simulink model "TorqueVectoring"  (R2024b)
settings: configuration reference "STM32H7_Config" (kept outside this file)
undefined symbols (not defined in the file): FStaticWeightFront, FStaticWeightRear, IYawInertia, lTrackWidth, lWheelbase, mCarMass, MMotorMaxAllowed, MMotorMinAllowed, MNominal, rGearboxRatio, rTyreRadius, tTorqueVectoringErrorCorrection, zCogHeight
libraries: simulink x10
settings Model: DataDictionary=Master_Dictionary.sldd  EnableAccessToBaseWorkspace=off  Creator=torni  LastModifiedBy=William
settings ConfigSetRef: SourceName=STM32H7_Config

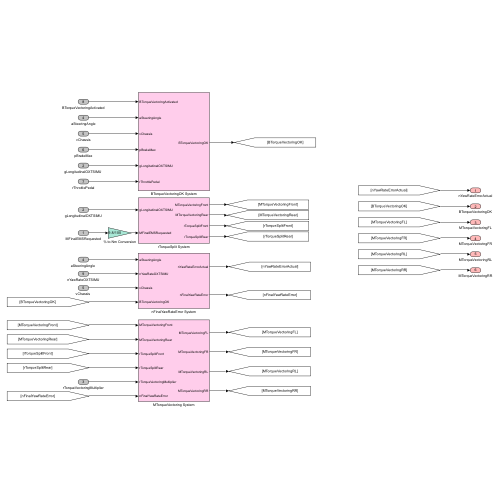
[thumbnail: Simulink's stored preview of the top-level diagram]
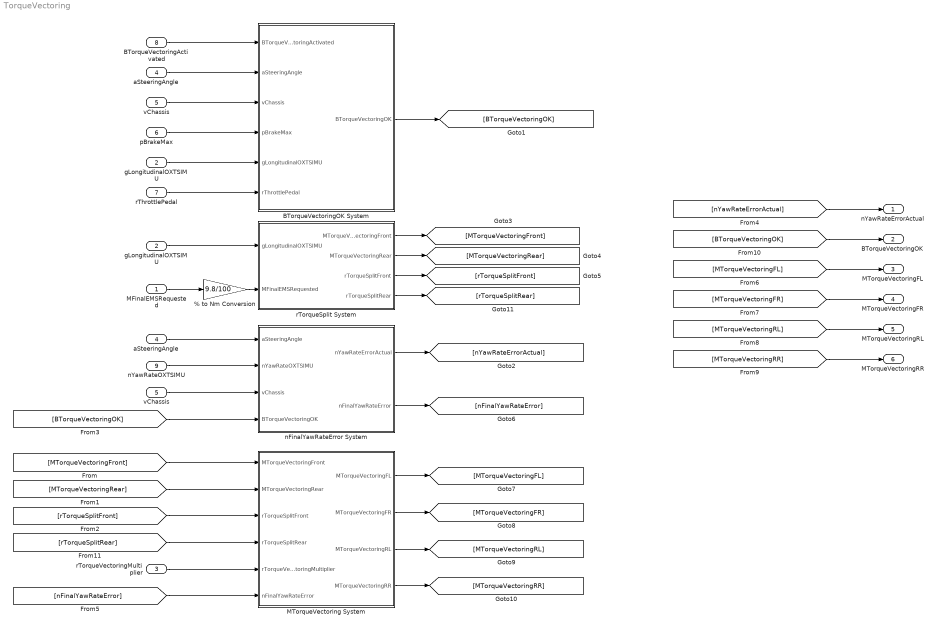
== system TorqueVectoring ==
  MFinalEMSRequested : Inport  OutDataTypeStr=double
  gLongitudinalOXTSIMU : Inport  Port=2  OutDataTypeStr=double
  rTorqueVectoringMultiplier : Inport  Port=3  OutDataTypeStr=double
  aSteeringAngle : Inport  Port=4  OutDataTypeStr=double
  vChassis : Inport  Port=5  OutDataTypeStr=double
  pBrakeMax : Inport  Port=6  OutDataTypeStr=double
  rThrottlePedal : Inport  Port=7  OutDataTypeStr=double
  BTorqueVectoringActivated : Inport  Port=8  OutDataTypeStr=boolean
  nYawRateOXTSIMU : Inport  Port=9  OutDataTypeStr=double
  % to Nm Conversion : Gain  Gain=9.8/100
  BTorqueVectoringOK System : Subsystem
  MTorqueVectoring System : Subsystem
  "aSteeringAngle " : InportShadow  Port=4  OutDataTypeStr=double
  "gLongitudinalOXTSIMU " : InportShadow  Port=2  OutDataTypeStr=double
  nFinalYawRateError System : Subsystem
  rTorqueSplit System : Subsystem
  "vChassis " : InportShadow  Port=5  OutDataTypeStr=double
  nYawRateErrorActual : Outport  OutDataTypeStr=double  VectorParamsAs1DForOutWhenUnconnected=off
  BTorqueVectoringOK : Outport  Port=2  OutDataTypeStr=boolean  VectorParamsAs1DForOutWhenUnconnected=off
  MTorqueVectoringFL : Outport  Port=3  OutDataTypeStr=double  VectorParamsAs1DForOutWhenUnconnected=off
  MTorqueVectoringFR : Outport  Port=4  OutDataTypeStr=double  VectorParamsAs1DForOutWhenUnconnected=off
  MTorqueVectoringRL : Outport  Port=5  OutDataTypeStr=double  VectorParamsAs1DForOutWhenUnconnected=off
  MTorqueVectoringRR : Outport  Port=6  OutDataTypeStr=double  VectorParamsAs1DForOutWhenUnconnected=off
  wires:
  rTorqueSplit System/2(MTorqueVectoringRear) -> [MTorqueVectoringRear]
  gLongitudinalOXTSIMU/1 -> rTorqueSplit System/1(gLongitudinalOXTSIMU)
  % to Nm Conversion/1 -> rTorqueSplit System/2(MFinalEMSRequested)
  MFinalEMSRequested/1 -> % to Nm Conversion/1
  rTorqueSplit System/1(MTorqueVectoringFront) -> [MTorqueVectoringFront]
  rTorqueSplit System/3(rTorqueSplitFront) -> [rTorqueSplitFront]
  [MTorqueVectoringFront] -> MTorqueVectoring System/1(MTorqueVectoringFront)
  [rTorqueSplitFront] -> MTorqueVectoring System/3(rTorqueSplitFront)
  BTorqueVectoringActivated/1 -> BTorqueVectoringOK System/1(BTorqueVectoringActivated)
  aSteeringAngle/1 -> BTorqueVectoringOK System/2(aSteeringAngle)
  vChassis/1 -> BTorqueVectoringOK System/3(vChassis)
  pBrakeMax/1 -> BTorqueVectoringOK System/4(pBrakeMax)
  "gLongitudinalOXTSIMU "/1 -> BTorqueVectoringOK System/5(gLongitudinalOXTSIMU)
  rThrottlePedal/1 -> BTorqueVectoringOK System/6(rThrottlePedal)
  BTorqueVectoringOK System/1(BTorqueVectoringOK) -> [BTorqueVectoringOK]
  rTorqueVectoringMultiplier/1 -> MTorqueVectoring System/5(rTorqueVectoringMultiplier)
  "aSteeringAngle "/1 -> nFinalYawRateError System/1(aSteeringAngle)
  nYawRateOXTSIMU/1 -> nFinalYawRateError System/2(nYawRateOXTSIMU)
  "vChassis "/1 -> nFinalYawRateError System/3(vChassis)
  [BTorqueVectoringOK] -> nFinalYawRateError System/4(BTorqueVectoringOK)
  nFinalYawRateError System/1(nYawRateErrorActual) -> [nYawRateErrorActual]
  nFinalYawRateError System/2(nFinalYawRateError) -> [nFinalYawRateError]
  [MTorqueVectoringRear] -> MTorqueVectoring System/2(MTorqueVectoringRear)
  [nFinalYawRateError] -> MTorqueVectoring System/6(nFinalYawRateError)
  MTorqueVectoring System/1(MTorqueVectoringFL) -> [MTorqueVectoringFL]
  MTorqueVectoring System/2(MTorqueVectoringFR) -> [MTorqueVectoringFR]
  MTorqueVectoring System/3(MTorqueVectoringRL) -> [MTorqueVectoringRL]
  MTorqueVectoring System/4(MTorqueVectoringRR) -> [MTorqueVectoringRR]
  [nYawRateErrorActual] -> nYawRateErrorActual/1
  [BTorqueVectoringOK] -> BTorqueVectoringOK/1
  [MTorqueVectoringFL] -> MTorqueVectoringFL/1
  [MTorqueVectoringFR] -> MTorqueVectoringFR/1
  [MTorqueVectoringRL] -> MTorqueVectoringRL/1
  [MTorqueVectoringRR] -> MTorqueVectoringRR/1
  rTorqueSplit System/4(rTorqueSplitRear) -> [rTorqueSplitRear]
  [rTorqueSplitRear] -> MTorqueVectoring System/4(rTorqueSplitRear)

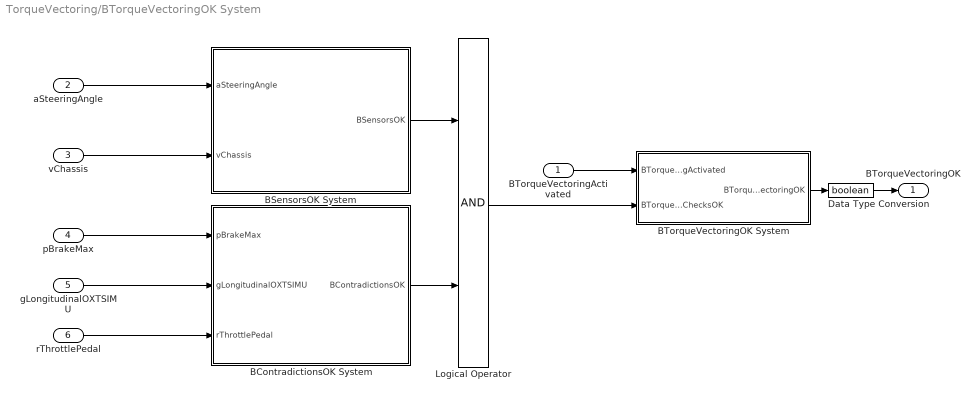
== system TorqueVectoring/BTorqueVectoringOK System ==
  BTorqueVectoringActivated : Inport  OutDataTypeStr=boolean
  aSteeringAngle : Inport  Port=2  OutDataTypeStr=double
  vChassis : Inport  Port=3  OutDataTypeStr=double
  pBrakeMax : Inport  Port=4  OutDataTypeStr=double
  gLongitudinalOXTSIMU : Inport  Port=5  OutDataTypeStr=double
  rThrottlePedal : Inport  Port=6  OutDataTypeStr=double
  BContradictionsOK System : Subsystem
  BSensorsOK System : Subsystem
  BTorqueVectoringOK System : Stateflow chart  TreatAsAtomicUnit=on
  Data Type Conversion : DataTypeConversion  OutDataTypeStr=boolean  SaturateOnIntegerOverflow=off  RndMeth=Floor
  Logical Operator : Logic  AllPortsSameDT=off  OutDataTypeStr=boolean
  BTorqueVectoringOK : Outport  OutDataTypeStr=boolean  VectorParamsAs1DForOutWhenUnconnected=off
  wires:
  pBrakeMax/1 -> BContradictionsOK System/1(pBrakeMax)
  rThrottlePedal/1 -> BContradictionsOK System/3(rThrottlePedal)
  Logical Operator/1 -> BTorqueVectoringOK System/2(BTorqueVectoringChecksOK)
  BTorqueVectoringOK System/1(BTorqueVectoringOK) -> Data Type Conversion/1
  BContradictionsOK System/1(BContradictionsOK) -> Logical Operator/2
  gLongitudinalOXTSIMU/1 -> BContradictionsOK System/2(gLongitudinalOXTSIMU)
  vChassis/1 -> BSensorsOK System/2(vChassis)
  BSensorsOK System/1(BSensorsOK) -> Logical Operator/1
  aSteeringAngle/1 -> BSensorsOK System/1(aSteeringAngle)
  BTorqueVectoringActivated/1 -> BTorqueVectoringOK System/1(BTorqueVectoringActivated)
  Data Type Conversion/1 -> BTorqueVectoringOK/1

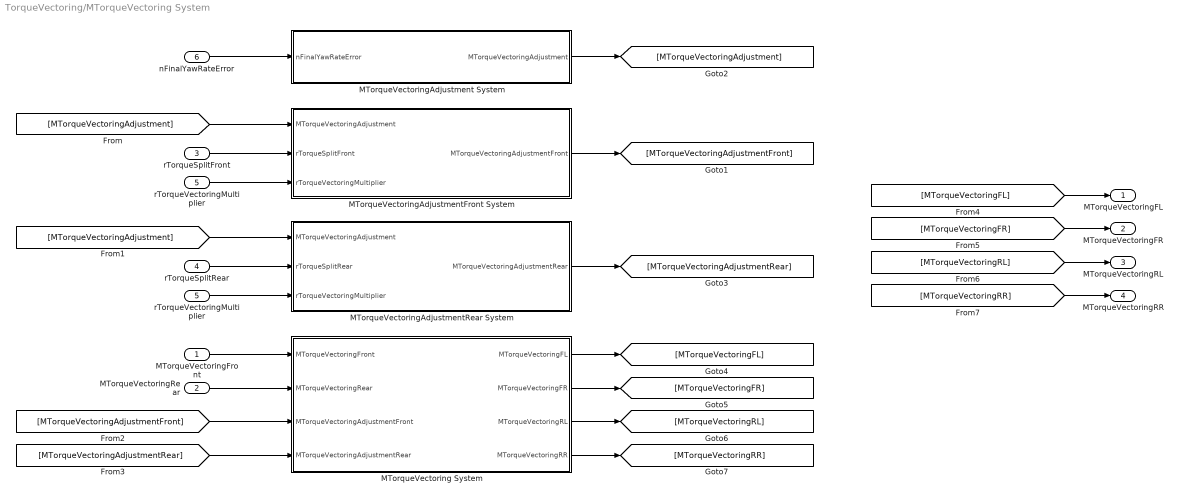
== system TorqueVectoring/MTorqueVectoring System ==
  MTorqueVectoringFront : Inport
  MTorqueVectoringRear : Inport  Port=2
  rTorqueSplitFront : Inport  Port=3  OutDataTypeStr=double
  rTorqueSplitRear : Inport  Port=4  OutDataTypeStr=double
  rTorqueVectoringMultiplier : Inport  Port=5  OutDataTypeStr=double
  nFinalYawRateError : Inport  Port=6  OutDataTypeStr=double
  MTorqueVectoring System : Subsystem
  MTorqueVectoringAdjustment System : Subsystem
  MTorqueVectoringAdjustmentFront System : Subsystem
  MTorqueVectoringAdjustmentRear System : Subsystem
  "rTorqueVectoringMultiplier " : InportShadow  Port=5  OutDataTypeStr=double
  MTorqueVectoringFL : Outport  OutDataTypeStr=double  VectorParamsAs1DForOutWhenUnconnected=off
  MTorqueVectoringFR : Outport  Port=2  OutDataTypeStr=double  VectorParamsAs1DForOutWhenUnconnected=off
  MTorqueVectoringRL : Outport  Port=3  OutDataTypeStr=double  VectorParamsAs1DForOutWhenUnconnected=off
  MTorqueVectoringRR : Outport  Port=4  OutDataTypeStr=double  VectorParamsAs1DForOutWhenUnconnected=off
  wires:
  nFinalYawRateError/1 -> MTorqueVectoringAdjustment System/1(nFinalYawRateError)
  MTorqueVectoringAdjustment System/1(MTorqueVectoringAdjustment) -> [MTorqueVectoringAdjustment]
  rTorqueSplitFront/1 -> MTorqueVectoringAdjustmentFront System/2(rTorqueSplitFront)
  [MTorqueVectoringAdjustment] -> MTorqueVectoringAdjustmentFront System/1(MTorqueVectoringAdjustment)
  rTorqueVectoringMultiplier/1 -> MTorqueVectoringAdjustmentFront System/3(rTorqueVectoringMultiplier)
  MTorqueVectoringAdjustmentFront System/1(MTorqueVectoringAdjustmentFront) -> [MTorqueVectoringAdjustmentFront]
  [MTorqueVectoringAdjustment] -> MTorqueVectoringAdjustmentRear System/1(MTorqueVectoringAdjustment)
  rTorqueSplitRear/1 -> MTorqueVectoringAdjustmentRear System/2(rTorqueSplitRear)
  "rTorqueVectoringMultiplier "/1 -> MTorqueVectoringAdjustmentRear System/3(rTorqueVectoringMultiplier)
  MTorqueVectoringAdjustmentRear System/1(MTorqueVectoringAdjustmentRear) -> [MTorqueVectoringAdjustmentRear]
  MTorqueVectoringFront/1 -> MTorqueVectoring System/1(MTorqueVectoringFront)
  MTorqueVectoringRear/1 -> MTorqueVectoring System/2(MTorqueVectoringRear)
  [MTorqueVectoringAdjustmentFront] -> MTorqueVectoring System/3(MTorqueVectoringAdjustmentFront)
  [MTorqueVectoringAdjustmentRear] -> MTorqueVectoring System/4(MTorqueVectoringAdjustmentRear)
  MTorqueVectoring System/1(MTorqueVectoringFL) -> [MTorqueVectoringFL]
  MTorqueVectoring System/2(MTorqueVectoringFR) -> [MTorqueVectoringFR]
  MTorqueVectoring System/3(MTorqueVectoringRL) -> [MTorqueVectoringRL]
  MTorqueVectoring System/4(MTorqueVectoringRR) -> [MTorqueVectoringRR]
  [MTorqueVectoringFL] -> MTorqueVectoringFL/1
  [MTorqueVectoringFR] -> MTorqueVectoringFR/1
  [MTorqueVectoringRL] -> MTorqueVectoringRL/1
  [MTorqueVectoringRR] -> MTorqueVectoringRR/1

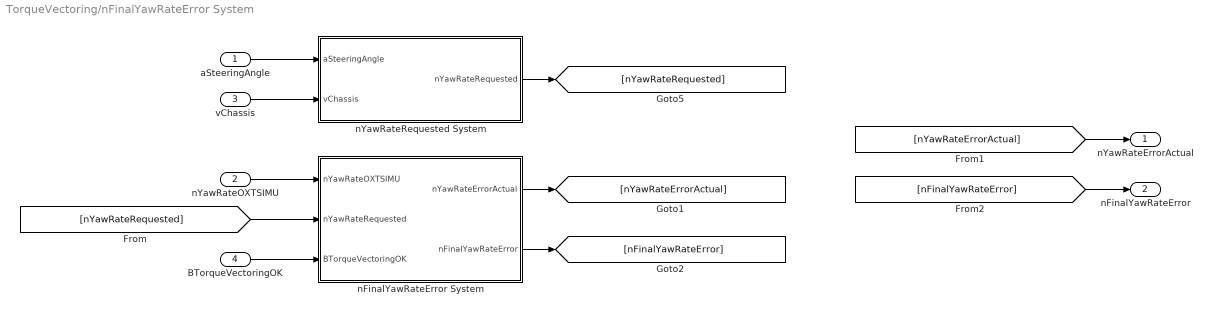
== system TorqueVectoring/nFinalYawRateError System ==
  aSteeringAngle : Inport  OutDataTypeStr=double
  nYawRateOXTSIMU : Inport  Port=2  OutDataTypeStr=double
  vChassis : Inport  Port=3  OutDataTypeStr=double
  BTorqueVectoringOK : Inport  Port=4  OutDataTypeStr=boolean
  nFinalYawRateError System : Subsystem
  nYawRateRequested System : Subsystem
  nYawRateErrorActual : Outport  OutDataTypeStr=double  VectorParamsAs1DForOutWhenUnconnected=off
  nFinalYawRateError : Outport  Port=2  OutDataTypeStr=double  VectorParamsAs1DForOutWhenUnconnected=off
  wires:
  aSteeringAngle/1 -> nYawRateRequested System/1(aSteeringAngle)
  vChassis/1 -> nYawRateRequested System/2(vChassis)
  nYawRateRequested System/1(nYawRateRequested) -> [nYawRateRequested]
  nYawRateOXTSIMU/1 -> nFinalYawRateError System/1(nYawRateOXTSIMU)
  [nYawRateRequested] -> nFinalYawRateError System/2(nYawRateRequested)
  BTorqueVectoringOK/1 -> nFinalYawRateError System/3(BTorqueVectoringOK)
  nFinalYawRateError System/1(nYawRateErrorActual) -> [nYawRateErrorActual]
  nFinalYawRateError System/2(nFinalYawRateError) -> [nFinalYawRateError]
  [nYawRateErrorActual] -> nYawRateErrorActual/1
  [nFinalYawRateError] -> nFinalYawRateError/1

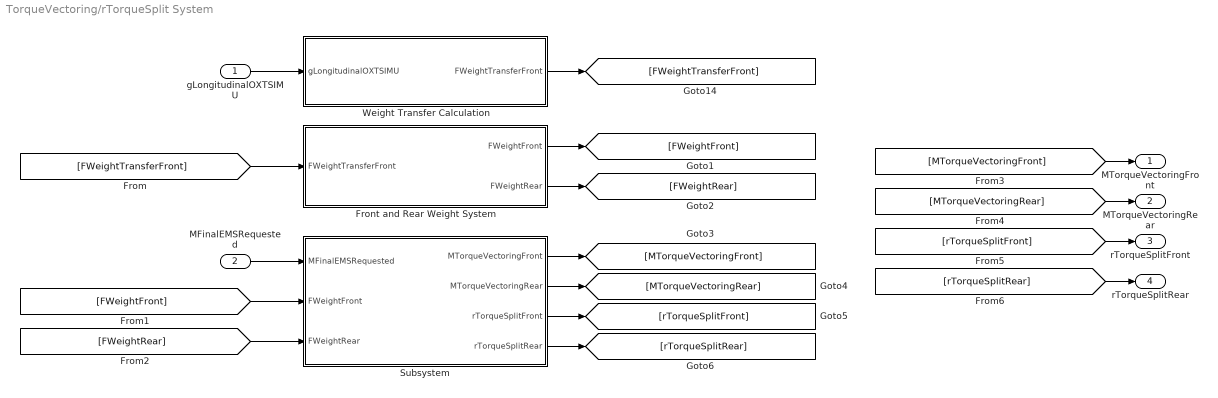
== system TorqueVectoring/rTorqueSplit System ==
  gLongitudinalOXTSIMU : Inport  OutDataTypeStr=double
  MFinalEMSRequested : Inport  Port=2  OutDataTypeStr=double
  Front and Rear Weight System : Subsystem
  Subsystem : Subsystem
  Weight Transfer Calculation : Subsystem
  MTorqueVectoringFront : Outport  OutDataTypeStr=double  VectorParamsAs1DForOutWhenUnconnected=off
  MTorqueVectoringRear : Outport  Port=2  OutDataTypeStr=double  VectorParamsAs1DForOutWhenUnconnected=off
  rTorqueSplitFront : Outport  Port=3  OutDataTypeStr=double  VectorParamsAs1DForOutWhenUnconnected=off
  rTorqueSplitRear : Outport  Port=4  OutDataTypeStr=double  VectorParamsAs1DForOutWhenUnconnected=off
  wires:
  Weight Transfer Calculation/1(FWeightTransferFront) -> [FWeightTransferFront]
  gLongitudinalOXTSIMU/1 -> Weight Transfer Calculation/1(gLongitudinalOXTSIMU)
  [FWeightTransferFront] -> Front and Rear Weight System/1(FWeightTransferFront)
  Front and Rear Weight System/1(FWeightFront) -> [FWeightFront]
  Front and Rear Weight System/2(FWeightRear) -> [FWeightRear]
  MFinalEMSRequested/1 -> Subsystem/1(MFinalEMSRequested)
  [FWeightFront] -> Subsystem/2(FWeightFront)
  [FWeightRear] -> Subsystem/3(FWeightRear)
  Subsystem/1(MTorqueVectoringFront) -> [MTorqueVectoringFront]
  Subsystem/2(MTorqueVectoringRear) -> [MTorqueVectoringRear]
  Subsystem/3(rTorqueSplitFront) -> [rTorqueSplitFront]
  [MTorqueVectoringFront] -> MTorqueVectoringFront/1
  [MTorqueVectoringRear] -> MTorqueVectoringRear/1
  [rTorqueSplitFront] -> rTorqueSplitFront/1
  Subsystem/4(rTorqueSplitRear) -> [rTorqueSplitRear]
  [rTorqueSplitRear] -> rTorqueSplitRear/1

== system TorqueVectoring/BTorqueVectoringOK System/BContradictionsOK System ==
  pBrakeMax : Inport  OutDataTypeStr=double
  gLongitudinalOXTSIMU : Inport  Port=2  OutDataTypeStr=double
  rThrottlePedal : Inport  Port=3  OutDataTypeStr=double
  Brake Contradiction : Subsystem
  Data Type Conversion : DataTypeConversion  OutDataTypeStr=boolean  SaturateOnIntegerOverflow=off  RndMeth=Floor
  Logical Operator : Logic  AllPortsSameDT=off  OutDataTypeStr=boolean
  Throttle Contradiction : Subsystem
  BContradictionsOK : Outport  OutDataTypeStr=boolean  VectorParamsAs1DForOutWhenUnconnected=off
  wires:
  Throttle Contradiction/1(BThrottleContradictionOK) -> Logical Operator/2
  Brake Contradiction/1(BBrakeContradictionOK) -> Logical Operator/1
  Logical Operator/1 -> Data Type Conversion/1
  pBrakeMax/1 -> Brake Contradiction/1(pBrakeMax)
  gLongitudinalOXTSIMU/1 -> Brake Contradiction/2(gLongitudinalOXTSIMU), Throttle Contradiction/1(gLongitudinalBoschIMU)
  rThrottlePedal/1 -> Throttle Contradiction/2(rThrottlePedal)
  Data Type Conversion/1 -> BContradictionsOK/1

== system TorqueVectoring/BTorqueVectoringOK System/BSensorsOK System ==
  aSteeringAngle : Inport  OutDataTypeStr=double
  vChassis : Inport  Port=2  OutDataTypeStr=double
  BSteeringAngleOK System : Subsystem
  BVelocityOK System : Subsystem
  Logical Operator : Logic  AllPortsSameDT=off  OutDataTypeStr=boolean
  BSensorsOK : Outport  OutDataTypeStr=boolean  VectorParamsAs1DForOutWhenUnconnected=off
  wires:
  BVelocityOK System/1(BVelocityOK) -> Logical Operator/1
  BSteeringAngleOK System/1(BSteeringAngleOK) -> Logical Operator/2
  Logical Operator/1 -> BSensorsOK/1
  vChassis/1 -> BVelocityOK System/1(vChassis)
  aSteeringAngle/1 -> BSteeringAngleOK System/1(aSteeringAngle)

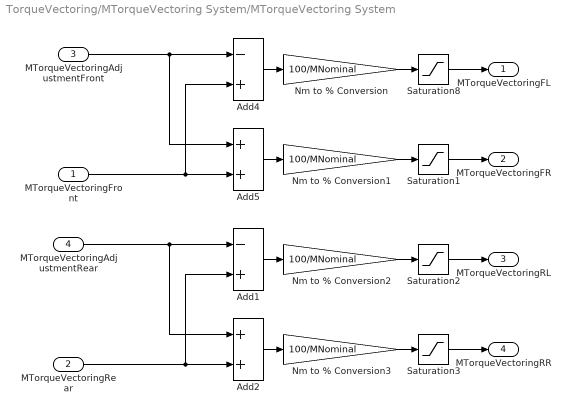
== system TorqueVectoring/MTorqueVectoring System/MTorqueVectoring System ==
  MTorqueVectoringFront : Inport  OutDataTypeStr=double
  MTorqueVectoringRear : Inport  Port=2  OutDataTypeStr=double
  MTorqueVectoringAdjustmentFront : Inport  Port=3  OutDataTypeStr=double
  MTorqueVectoringAdjustmentRear : Inport  Port=4  OutDataTypeStr=double
  Add1 : Sum  Inputs=-+
  Add2 : Sum
  Add4 : Sum  Inputs=-+
  Add5 : Sum
  Nm to % Conversion{,1..3} (4 alike) : Gain  Gain=100/MNominal
  Saturation{1..3,8} (4 alike) : Saturate  UpperLimit=MMotorMaxAllowed  LowerLimit=MMotorMinAllowed
  MTorqueVectoringFL : Outport  OutDataTypeStr=double  VectorParamsAs1DForOutWhenUnconnected=off
  MTorqueVectoringFR : Outport  Port=2  OutDataTypeStr=double  VectorParamsAs1DForOutWhenUnconnected=off
  MTorqueVectoringRL : Outport  Port=3  OutDataTypeStr=double  VectorParamsAs1DForOutWhenUnconnected=off
  MTorqueVectoringRR : Outport  Port=4  OutDataTypeStr=double  VectorParamsAs1DForOutWhenUnconnected=off
  wires:
  MTorqueVectoringAdjustmentFront/1 -> Add5/1, Add4/1
  Add4/1 -> Nm to % Conversion/1
  Add5/1 -> Nm to % Conversion1/1
  Saturation1/1 -> MTorqueVectoringFR/1
  Nm to % Conversion/1 -> Saturation8/1
  Saturation8/1 -> MTorqueVectoringFL/1
  MTorqueVectoringFront/1 -> Add4/2, Add5/2
  Nm to % Conversion1/1 -> Saturation1/1
  Nm to % Conversion3/1 -> Saturation3/1
  MTorqueVectoringRear/1 -> Add2/2, Add1/2
  Saturation2/1 -> MTorqueVectoringRL/1
  Nm to % Conversion2/1 -> Saturation2/1
  Saturation3/1 -> MTorqueVectoringRR/1
  Add2/1 -> Nm to % Conversion3/1
  Add1/1 -> Nm to % Conversion2/1
  MTorqueVectoringAdjustmentRear/1 -> Add1/1, Add2/1

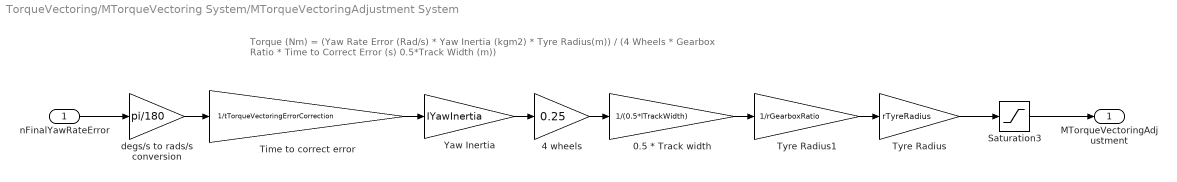
== system TorqueVectoring/MTorqueVectoring System/MTorqueVectoringAdjustment System ==
  note: Torque (Nm) = (Yaw Rate Error (Rad/s) * Yaw Inertia (kgm2) * Tyre Radius(m)) / (4 Wheels * Gearbox Ratio * Time to Correct Error (s) 0.5*Track Width (m))
  nFinalYawRateError : Inport  OutDataTypeStr=double
  0.5 * Track width : Gain  Gain=1/(0.5*lTrackWidth)
  4 wheels : Gain  Gain=0.25
  Saturation3 : Saturate  UpperLimit=10  LowerLimit=-10
  Time to correct error : Gain  Gain=1/tTorqueVectoringErrorCorrection
  Tyre Radius : Gain  Gain=rTyreRadius
  Tyre Radius1 : Gain  Gain=1/rGearboxRatio
  Yaw Inertia : Gain  Gain=IYawInertia
  degs/s to rads/s conversion : Gain  Gain=pi/180
  MTorqueVectoringAdjustment : Outport  OutDataTypeStr=double  VectorParamsAs1DForOutWhenUnconnected=off
  wires:
  Time to correct error/1 -> Yaw Inertia/1
  0.5 * Track width/1 -> Tyre Radius1/1
  degs/s to rads/s conversion/1 -> Time to correct error/1
  4 wheels/1 -> 0.5 * Track width/1
  Yaw Inertia/1 -> 4 wheels/1
  Tyre Radius/1 -> Saturation3/1
  nFinalYawRateError/1 -> degs/s to rads/s conversion/1
  Saturation3/1 -> MTorqueVectoringAdjustment/1
  Tyre Radius1/1 -> Tyre Radius/1

== system TorqueVectoring/MTorqueVectoring System/MTorqueVectoringAdjustmentFront System ==
  MTorqueVectoringAdjustment : Inport  OutDataTypeStr=double
  rTorqueSplitFront : Inport  Port=2  OutDataTypeStr=double
  rTorqueVectoringMultiplier : Inport  Port=3  OutDataTypeStr=double
  Multiply : Product  Inputs=3
  MTorqueVectoringAdjustmentFront : Outport  OutDataTypeStr=double  VectorParamsAs1DForOutWhenUnconnected=off
  wires:
  rTorqueSplitFront/1 -> Multiply/2
  MTorqueVectoringAdjustment/1 -> Multiply/1
  rTorqueVectoringMultiplier/1 -> Multiply/3
  Multiply/1 -> MTorqueVectoringAdjustmentFront/1

== system TorqueVectoring/MTorqueVectoring System/MTorqueVectoringAdjustmentRear System ==
  MTorqueVectoringAdjustment : Inport  OutDataTypeStr=double
  rTorqueSplitRear : Inport  Port=2  OutDataTypeStr=double
  rTorqueVectoringMultiplier : Inport  Port=3  OutDataTypeStr=double
  Multiply : Product  Inputs=3
  MTorqueVectoringAdjustmentRear : Outport  OutDataTypeStr=double  VectorParamsAs1DForOutWhenUnconnected=off
  wires:
  Multiply/1 -> MTorqueVectoringAdjustmentRear/1
  rTorqueVectoringMultiplier/1 -> Multiply/3
  MTorqueVectoringAdjustment/1 -> Multiply/1
  rTorqueSplitRear/1 -> Multiply/2

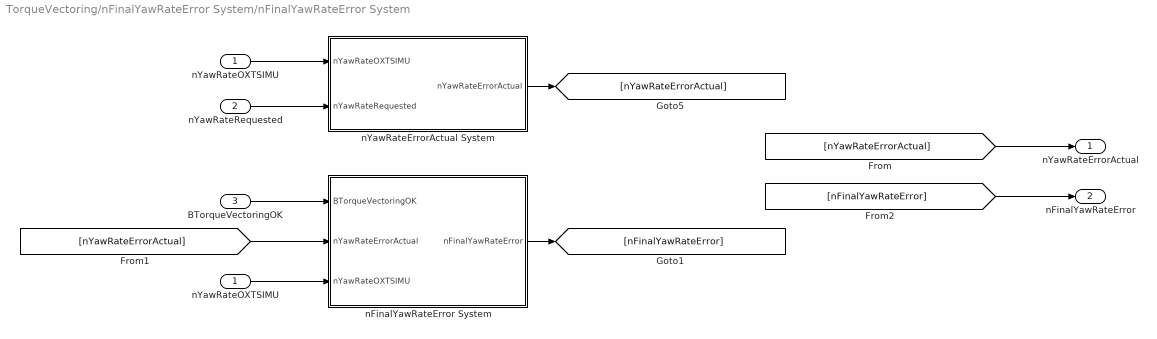
== system TorqueVectoring/nFinalYawRateError System/nFinalYawRateError System ==
  nYawRateOXTSIMU : Inport  OutDataTypeStr=double
  nYawRateRequested : Inport  Port=2  OutDataTypeStr=double
  BTorqueVectoringOK : Inport  Port=3  OutDataTypeStr=boolean
  nFinalYawRateError System : Subsystem
  nYawRateErrorActual System : Subsystem
  "nYawRateOXTSIMU " : InportShadow  OutDataTypeStr=double
  nYawRateErrorActual : Outport  OutDataTypeStr=double  VectorParamsAs1DForOutWhenUnconnected=off
  nFinalYawRateError : Outport  Port=2  OutDataTypeStr=double  VectorParamsAs1DForOutWhenUnconnected=off
  wires:
  nYawRateOXTSIMU/1 -> nYawRateErrorActual System/1(nYawRateOXTSIMU)
  nYawRateRequested/1 -> nYawRateErrorActual System/2(nYawRateRequested)
  nYawRateErrorActual System/1(nYawRateErrorActual) -> [nYawRateErrorActual]
  BTorqueVectoringOK/1 -> nFinalYawRateError System/1(BTorqueVectoringOK)
  "nYawRateOXTSIMU "/1 -> nFinalYawRateError System/3(nYawRateOXTSIMU)
  [nYawRateErrorActual] -> nFinalYawRateError System/2(nYawRateErrorActual)
  [nYawRateErrorActual] -> nYawRateErrorActual/1
  nFinalYawRateError System/1(nFinalYawRateError) -> [nFinalYawRateError]
  [nFinalYawRateError] -> nFinalYawRateError/1

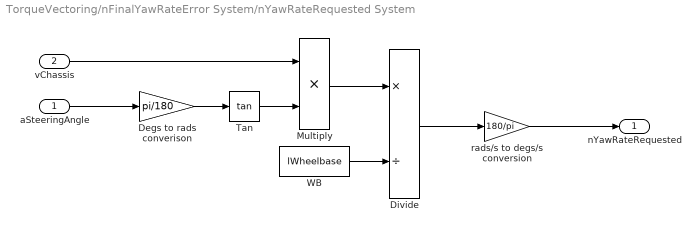
== system TorqueVectoring/nFinalYawRateError System/nYawRateRequested System ==
  aSteeringAngle : Inport  OutDataTypeStr=double
  vChassis : Inport  Port=2  OutDataTypeStr=double
  Degs to rads converison : Gain  Gain=pi/180
  Divide : Product  Inputs=*/  RndMeth=Zero  SaturateOnIntegerOverflow=on
  Multiply : Product
  Tan : Trigonometry  Operator=tan
  WB : Constant  Value=lWheelbase
  rads/s to degs/s conversion : Gain  Gain=180/pi
  nYawRateRequested : Outport  OutDataTypeStr=double  VectorParamsAs1DForOutWhenUnconnected=off
  wires:
  WB/1 -> Divide/2
  aSteeringAngle/1 -> Degs to rads converison/1
  Divide/1 -> rads/s to degs/s conversion/1
  rads/s to degs/s conversion/1 -> nYawRateRequested/1
  Tan/1 -> Multiply/2
  vChassis/1 -> Multiply/1
  Multiply/1 -> Divide/1
  Degs to rads converison/1 -> Tan/1

== system TorqueVectoring/rTorqueSplit System/Front and Rear Weight System ==
  FWeightTransferFront : Inport  OutDataTypeStr=double
  Add : Sum
  Add1 : Sum  Inputs=+-
  Constant : Constant  Value=FStaticWeightFront
  Constant1 : Constant  Value=FStaticWeightRear
  FWeightFront : Outport  OutDataTypeStr=double  VectorParamsAs1DForOutWhenUnconnected=off
  FWeightRear : Outport  Port=2  OutDataTypeStr=double  VectorParamsAs1DForOutWhenUnconnected=off
  wires:
  Add1/1 -> FWeightRear/1
  FWeightTransferFront/1 -> Add1/2, Add/2
  Add/1 -> FWeightFront/1
  Constant1/1 -> Add1/1
  Constant/1 -> Add/1

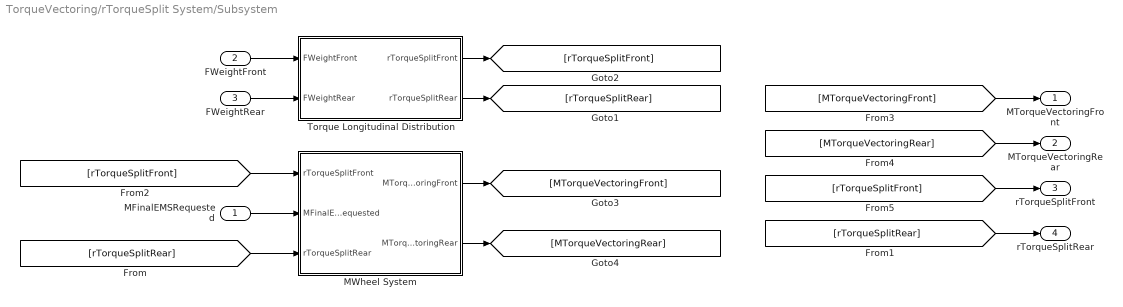
== system TorqueVectoring/rTorqueSplit System/Subsystem ==
  MFinalEMSRequested : Inport  OutDataTypeStr=double
  FWeightFront : Inport  Port=2  OutDataTypeStr=double
  FWeightRear : Inport  Port=3  OutDataTypeStr=double
  MWheel System : Subsystem
  Torque Longitudinal Distribution : MATLAB Function  TreatAsAtomicUnit=on
  MTorqueVectoringFront : Outport  OutDataTypeStr=double  VectorParamsAs1DForOutWhenUnconnected=off
  MTorqueVectoringRear : Outport  Port=2  OutDataTypeStr=double  VectorParamsAs1DForOutWhenUnconnected=off
  rTorqueSplitFront : Outport  Port=3  OutDataTypeStr=double  VectorParamsAs1DForOutWhenUnconnected=off
  rTorqueSplitRear : Outport  Port=4  OutDataTypeStr=double  VectorParamsAs1DForOutWhenUnconnected=off
  wires:
  FWeightRear/1 -> Torque Longitudinal Distribution/2(FWeightRear)
  FWeightFront/1 -> Torque Longitudinal Distribution/1(FWeightFront)
  Torque Longitudinal Distribution/1(rTorqueSplitFront) -> [rTorqueSplitFront]
  Torque Longitudinal Distribution/2(rTorqueSplitRear) -> [rTorqueSplitRear]
  MFinalEMSRequested/1 -> MWheel System/2(MFinalEMSRequested)
  [rTorqueSplitFront] -> MWheel System/1(rTorqueSplitFront)
  [rTorqueSplitRear] -> MWheel System/3(rTorqueSplitRear)
  [rTorqueSplitFront] -> rTorqueSplitFront/1
  MWheel System/1(MTorqueVectoringFront) -> [MTorqueVectoringFront]
  [MTorqueVectoringFront] -> MTorqueVectoringFront/1
  MWheel System/2(MTorqueVectoringRear) -> [MTorqueVectoringRear]
  [MTorqueVectoringRear] -> MTorqueVectoringRear/1
  [rTorqueSplitRear] -> rTorqueSplitRear/1

== system TorqueVectoring/rTorqueSplit System/Weight Transfer Calculation ==
  note: Weight Transfer Load = (Acceleration * Mass * CoG Height) / Wheelbase
  gLongitudinalOXTSIMU : Inport  OutDataTypeStr=double
  1/Wheelbase : Gain  Gain=1/lWheelbase
  CoG Height : Gain  Gain=zCogHeight
  Mass : Gain  Gain=mCarMass
  Negative : Gain  Gain=-1
  FWeightTransferFront : Outport  OutDataTypeStr=double  VectorParamsAs1DForOutWhenUnconnected=off
  wires:
  1/Wheelbase/1 -> FWeightTransferFront/1
  Negative/1 -> Mass/1
  Mass/1 -> CoG Height/1
  gLongitudinalOXTSIMU/1 -> Negative/1
  CoG Height/1 -> 1/Wheelbase/1

== system TorqueVectoring/BTorqueVectoringOK System/BContradictionsOK System/Brake Contradiction ==
  pBrakeMax : Inport  OutDataTypeStr=double
  gLongitudinalOXTSIMU : Inport  Port=2  OutDataTypeStr=double
  Compare To Constant : simulink/Logic and Bit Operations/Compare To Constant  relop=>  const=10  OutDataTypeStr=boolean
  Compare To Constant1 : simulink/Logic and Bit Operations/Compare To Constant  relop=>  const=5  OutDataTypeStr=boolean
  Logical Operator1 : Logic  Operator=NAND  AllPortsSameDT=off  OutDataTypeStr=boolean
  BBrakeContradictionOK : Outport  OutDataTypeStr=boolean  VectorParamsAs1DForOutWhenUnconnected=off
  wires:
  Logical Operator1/1 -> BBrakeContradictionOK/1
  gLongitudinalOXTSIMU/1 -> Compare To Constant1/1
  Compare To Constant1/1 -> Logical Operator1/2
  Compare To Constant/1 -> Logical Operator1/1
  pBrakeMax/1 -> Compare To Constant/1

== system TorqueVectoring/BTorqueVectoringOK System/BContradictionsOK System/Throttle Contradiction ==
  gLongitudinalBoschIMU : Inport  OutDataTypeStr=double
  rThrottlePedal : Inport  Port=2  OutDataTypeStr=double
  Compare To Constant : simulink/Logic and Bit Operations/Compare To Constant  relop=>  const=80  OutDataTypeStr=boolean
  Compare To Constant1 : simulink/Logic and Bit Operations/Compare To Constant  relop=<  const=-5  OutDataTypeStr=boolean
  Logical Operator1 : Logic  Operator=NAND  AllPortsSameDT=off  OutDataTypeStr=boolean
  BThrottleContradictionOK : Outport  OutDataTypeStr=boolean  VectorParamsAs1DForOutWhenUnconnected=off
  wires:
  Logical Operator1/1 -> BThrottleContradictionOK/1
  rThrottlePedal/1 -> Compare To Constant/1
  Compare To Constant/1 -> Logical Operator1/1
  Compare To Constant1/1 -> Logical Operator1/2
  gLongitudinalBoschIMU/1 -> Compare To Constant1/1

== system TorqueVectoring/BTorqueVectoringOK System/BSensorsOK System/BSteeringAngleOK System ==
  aSteeringAngle : Inport  OutDataTypeStr=double
  Compare To Constant : simulink/Logic and Bit Operations/Compare To Constant  relop=>  const=-29  OutDataTypeStr=boolean
  Compare To Constant1 : simulink/Logic and Bit Operations/Compare To Constant  relop=<  const=29  OutDataTypeStr=boolean
  Logical Operator : Logic  AllPortsSameDT=off  OutDataTypeStr=boolean
  BSteeringAngleOK : Outport  OutDataTypeStr=boolean  VectorParamsAs1DForOutWhenUnconnected=off
  wires:
  Logical Operator/1 -> BSteeringAngleOK/1
  aSteeringAngle/1 -> Compare To Constant/1, Compare To Constant1/1
  Compare To Constant/1 -> Logical Operator/1
  Compare To Constant1/1 -> Logical Operator/2

== system TorqueVectoring/BTorqueVectoringOK System/BSensorsOK System/BVelocityOK System ==
  vChassis : Inport  OutDataTypeStr=double
  Compare To Constant : simulink/Logic and Bit Operations/Compare To Constant  relop=>  const=-2  OutDataTypeStr=boolean
  Compare To Constant1 : simulink/Logic and Bit Operations/Compare To Constant  relop=<  const=31  OutDataTypeStr=boolean
  Logical Operator : Logic  AllPortsSameDT=off  OutDataTypeStr=boolean
  BVelocityOK : Outport  OutDataTypeStr=boolean  VectorParamsAs1DForOutWhenUnconnected=off
  wires:
  Compare To Constant/1 -> Logical Operator/2
  Compare To Constant1/1 -> Logical Operator/1
  Logical Operator/1 -> BVelocityOK/1
  vChassis/1 -> Compare To Constant1/1, Compare To Constant/1

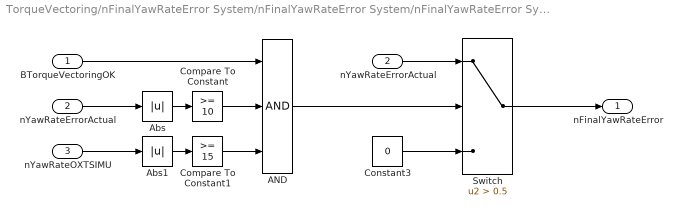
== system TorqueVectoring/nFinalYawRateError System/nFinalYawRateError System/nFinalYawRateError System ==
  BTorqueVectoringOK : Inport  OutDataTypeStr=boolean
  nYawRateErrorActual : Inport  Port=2  OutDataTypeStr=double
  nYawRateOXTSIMU : Inport  Port=3  OutDataTypeStr=double
  AND : Logic  Inputs=3  AllPortsSameDT=off  OutDataTypeStr=boolean
  Abs : Abs  SaturateOnIntegerOverflow=off
  Abs1 : Abs  SaturateOnIntegerOverflow=off
  Compare To Constant : simulink/Logic and Bit Operations/Compare To Constant  relop=>=  const=10  OutDataTypeStr=boolean
  Compare To Constant1 : simulink/Logic and Bit Operations/Compare To Constant  relop=>=  const=15  OutDataTypeStr=boolean
  Constant3 : Constant  Value=0
  Switch : Switch  Criteria=u2 > Threshold  Threshold=0.5  SaturateOnIntegerOverflow=off  InputSameDT=off
  "nYawRateErrorActual " : InportShadow  Port=2  OutDataTypeStr=double
  nFinalYawRateError : Outport  OutDataTypeStr=double  VectorParamsAs1DForOutWhenUnconnected=off
  wires:
  Abs1/1 -> Compare To Constant1/1
  Compare To Constant1/1 -> AND/3
  nYawRateOXTSIMU/1 -> Abs1/1
  "nYawRateErrorActual "/1 -> Switch/1
  Constant3/1 -> Switch/3
  AND/1 -> Switch/2
  Compare To Constant/1 -> AND/2
  nYawRateErrorActual/1 -> Abs/1
  Abs/1 -> Compare To Constant/1
  BTorqueVectoringOK/1 -> AND/1
  Switch/1 -> nFinalYawRateError/1

== system TorqueVectoring/nFinalYawRateError System/nFinalYawRateError System/nYawRateErrorActual System ==
  nYawRateOXTSIMU : Inport  OutDataTypeStr=double
  nYawRateRequested : Inport  Port=2  OutDataTypeStr=double
  Subtract : Sum  Inputs=-+
  nYawRateErrorActual : Outport  OutDataTypeStr=double  VectorParamsAs1DForOutWhenUnconnected=off
  wires:
  nYawRateOXTSIMU/1 -> Subtract/1
  nYawRateRequested/1 -> Subtract/2
  Subtract/1 -> nYawRateErrorActual/1

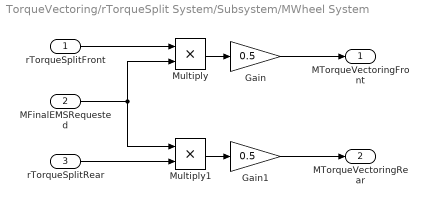
== system TorqueVectoring/rTorqueSplit System/Subsystem/MWheel System ==
  rTorqueSplitFront : Inport  OutDataTypeStr=double
  MFinalEMSRequested : Inport  Port=2  OutDataTypeStr=double
  rTorqueSplitRear : Inport  Port=3  OutDataTypeStr=double
  Gain : Gain  Gain=0.5
  Gain1 : Gain  Gain=0.5
  Multiply : Product
  Multiply1 : Product
  MTorqueVectoringFront : Outport  OutDataTypeStr=double  VectorParamsAs1DForOutWhenUnconnected=off
  MTorqueVectoringRear : Outport  Port=2  OutDataTypeStr=double  VectorParamsAs1DForOutWhenUnconnected=off
  wires:
  Multiply1/1 -> Gain1/1
  Gain/1 -> MTorqueVectoringFront/1
  Gain1/1 -> MTorqueVectoringRear/1
  MFinalEMSRequested/1 -> Multiply1/1, Multiply/2
  rTorqueSplitRear/1 -> Multiply1/2
  Multiply/1 -> Gain/1
  rTorqueSplitFront/1 -> Multiply/1

== stateflow chart TorqueVectoring/BTorqueVectoringOK System/BTorqueVectoringOK System ==
  state StartTV1
    BTorqueVectoringOK=1
  state StopTV
    BTorqueVectoringOK = 0
  StartTV1 -> StopTV : [BTorqueVectoringChecksOK<0.5]
  (default) -> StartTV1
  StopTV -> StartTV1 : [BTorqueVectoringActivated<0.5]
  data: BTorqueVectoringActivated input boolean; BTorqueVectoringChecksOK input boolean; BTorqueVectoringOK output double

== matlab function TorqueVectoring/rTorqueSplit System/Subsystem/Torque Longitudinal Distribution ==
  data: FWeightFront input; rTorqueSplitFront output; FWeightRear input; rTorqueSplitRear output
function [rTorqueSplitFront,rTorqueSplitRear]= fcn(FWeightFront, FWeightRear)
rTorqueSplitFront = FWeightFront/(FWeightFront + FWeightRear);
rTorqueSplitRear = FWeightRear/(FWeightFront + FWeightRear);
